simulink model "group5_A2finalmodel"  (R2023a)
settings: Solver=FixedStepAuto  StartTime=0.0  StopTime=10.0  FixedStep=1e-3  RelTol=1e-3  EnableMultiTasking=on
undefined symbols (not defined in the file): A0, A1, D0, D1, D10, D11, D12, D13, D2, D3, D4, D5, D6, D7, D8, D9, PTA0, PTA1, PTA2, PTB2, PTB23, PTB3, PTB9, PTC16, PTC17, PTC2, PTC3, PTC4, PTD0, PTD1, PTD2, PTD3
libraries: frdmk64flib x19, etargetslib x4, dspstat3 x1
settings Model: ExtModeTrigDuration=5  Creator=josep  LastModifiedBy=alast
settings SolverCC: AlgebraicLoopSolver=TrustRegion
settings OptimizationCC: EnhancedBackFolding=on  PassReuseOutputArgsAs=Individual arguments  ZeroExternalMemoryAtStartup=off  ZeroInternalMemoryAtStartup=off  MaxStackSize=64  OptimizeBlockOrder=speed  DifferentSizesBufferReuse=on  OptimizationCustomize=off  EfficientTunableParamExpr=on
settings DebuggingCC: ParameterTunabilityLossMsg=error
settings HardwareCC: ProdBitPerPointer=32  ProdBitPerSizeT=32  ProdBitPerPtrDiffT=32  ProdLargestAtomicInteger=Long  ProdLargestAtomicFloat=Double  ProdWordSize=32  ProdHWDeviceType=ARM Compatible->ARM Cortex
settings SFSimCC: MATLABDynamicMemAlloc=off
settings RTWCC: Description=Embedded Coder  SystemTargetFile=ert.tlc  HardwareBoard=NXP FRDM-K64F  TLCOptions="-aInlineSetEventsForThisBaseRateFcn=TLC_FALSE -aSuppressMultiTaskScheduler=TLC_FALSE  -aRateBasedStepFcn=0"  TemplateMakefile=ert_default_tmf  Toolchain=GNU Tools for ARM Embedded Processors
settings CodeAppCC: ForceParamTrailComments=on  IgnoreCustomStorageClasses=off  OperatorAnnotations=on  SimulinkDataObjDesc=on  SFDataObjDesc=on  InsertBlockDesc=on
settings ERTTargetCC: ExtModeTransport=4  ExtModeMexFile=sendToCommService

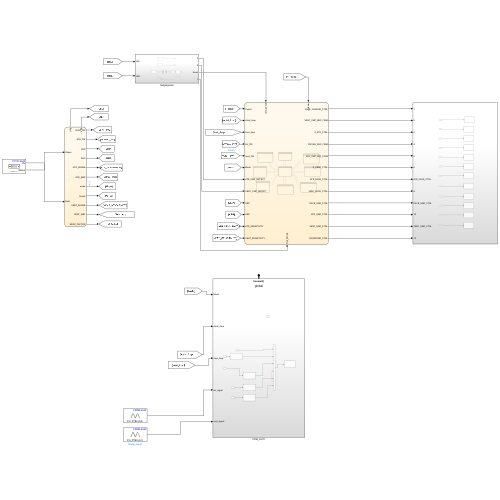
[thumbnail: Simulink's stored preview of the top-level diagram]
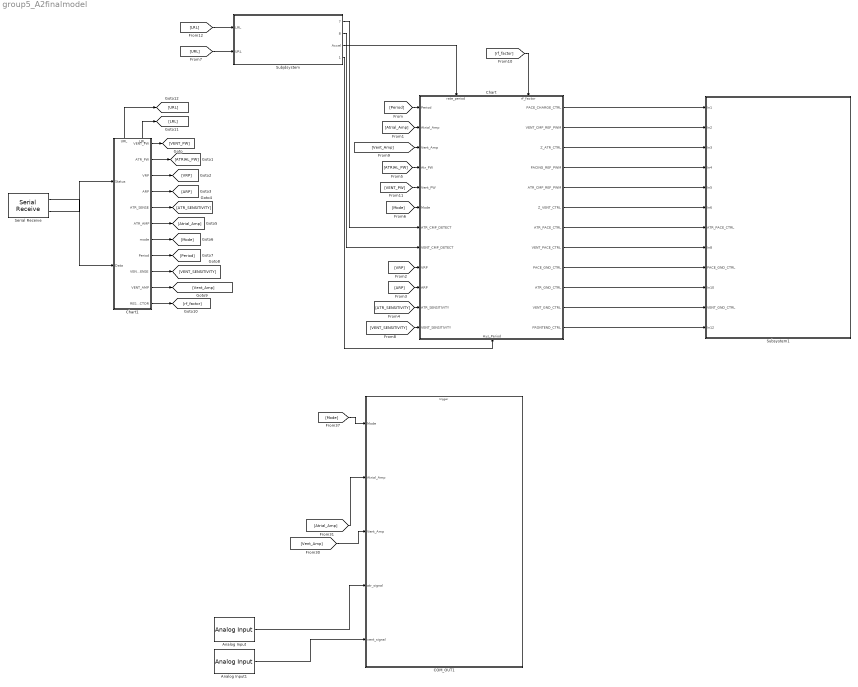
== system group5_A2finalmodel ==
  Analog Input : frdmk64flib/Analog Input  Whichpin=PTB2 (A0)  SampleTime=-1
  Analog Input1 : frdmk64flib/Analog Input  Whichpin=PTB3 (A1)  SampleTime=-1
  COM_OUT1 : Subsystem  TreatAsAtomicUnit=on
  Chart : Stateflow chart  TreatAsAtomicUnit=on
      settings: PortSchema="{\"entries\":[{\"content\":{\"sides\":[{\"content\":{\"connectorIds\":[\"In8\",\"In4\",\"In5\",\"In6\",\"In7\",\"In9\",\"In10\",\"In11\",\"In12\",\"In13\",\"In14\",\"In15\"]},\"type\":\"ConnectorPlacement.EquallySpacedRectSide\",\"uuid\":\"6343ef83-1ce8-46c7-8622-1dca0f09a909\"},{\"content\":{\"connectorIds\":[\"Out1\",\"Out2\",\"Out3\",\"Out4\",\"Out5\",\"Out6\",\"Out7\",\"Out8\",\"Out9\",\"Out10\",\"Out11\",\"Out12\"],\"side\":\"RIGHT\"},\"type\":\"ConnectorPlacement.EquallySpacedRectSide\",\"uuid\":\"7d8c9973-a2ea-42d1-99a2-efee47476445\"},{\"content\":{\"connectorIds\":[\"In1\",\"In2\"],\"side\":\"TOP\"},\"type\":\"ConnectorPlacement.EquallySpacedRectSide\",\"uuid\":\"d6f36041-fe62-4fd0-b92e-ddcbd2ff161d\"},{\"content\":{\"connectorIds\":[\"In3\"],\"side\":\"BOTTOM\"},\"type\":\"ConnectorPlacement.EquallySpacedRectSide\",\"uuid\":\"9ef693f9-8331-444a-9668-ba4dbf8aea62\"}]},\"type\":\"ConnectorPlacement.EquallySpacedConnector\",\"uuid\":\"1488a652-70a0-4b94-9610-167d4f46302b\"}],\"packageUris\":[\"http://schema.mathworks.com/mf0/Connector/R2020b\"],\"version\":\"1.0\"}"
  Chart1 : Stateflow chart  TreatAsAtomicUnit=on
      settings: PortSchema="{\"entries\":[{\"content\":{\"sides\":[{\"content\":{\"connectorIds\":[\"In1\",\"In2\"]},\"type\":\"ConnectorPlacement.EquallySpacedRectSide\",\"uuid\":\"8fb2c45e-5549-4401-9c79-42eba0e918c6\"},{\"content\":{\"connectorIds\":[\"Out3\",\"Out4\",\"Out5\",\"Out6\",\"Out7\",\"Out8\",\"Out9\",\"Out10\",\"Out11\",\"Out12\",\"Out13\"],\"side\":\"RIGHT\"},\"type\":\"ConnectorPlacement.EquallySpacedRectSide\",\"uuid\":\"7f0c3680-1cc1-4ed2-8a94-80b3abd25fe2\"},{\"content\":{\"connectorIds\":[\"Out1\",\"Out2\"],\"side\":\"TOP\"},\"type\":\"ConnectorPlacement.EquallySpacedRectSide\",\"uuid\":\"e6a4cd4f-b629-40f1-b56f-49c003080cda\"}]},\"type\":\"ConnectorPlacement.EquallySpacedConnector\",\"uuid\":\"c978f693-ab67-4a6f-917b-57d5c3fb90c1\"}],\"packageUris\":[\"http://schema.mathworks.com/mf0/Connector/R2020b\"],\"version\":\"1.0\"}"
  Serial Receive : frdmk64flib/Serial Receive  SCIModule=0  Baudrate=uint32(9600)  Parity=None  StopBits=1  HardwareFlowControl=None  ByteOrder=LittleEndian  DataType=uint8  DataLength=34  BlockingMode=off  OutputStatus=on  SampleTime=-1
  Subjdsystem : Subsystem
  Subsystem1 : Subsystem
  wires:
  Subjdsystem/1(7) -> Chart/10(ATR_CMP_DETECT)
  Subjdsystem/2(8) -> Chart/11(VENT_CMP_DETECT)
  Subjdsystem/3(Accel) -> Chart/1(rate_period)
  Chart/6(Z_VENT_CTRL) -> Subsystem1/6(In6)
  Chart/5(ATR_CMP_REF_PWM) -> Subsystem1/5(In5)
  Chart/4(PACING_REF_PWM) -> Subsystem1/4(In4)
  Chart/3(Z_ATR_CTRL) -> Subsystem1/3(In3)
  Chart/2(VENT_CMP_REF_PWM) -> Subsystem1/2(In2)
  Chart/7(ATR_PACE_CTRL) -> Subsystem1/7(ATR_PACE_CTRL)
  Chart/8(VENT_PACE_CTRL) -> Subsystem1/8(In8)
  Chart/9(PACE_GND_CTRL) -> Subsystem1/9(PACE_GND_CTRL)
  Chart/10(ATR_GND_CTRL) -> Subsystem1/10(In10)
  Chart/11(VENT_GND_CTRL) -> Subsystem1/11(VENT_GND_CTRL)
  Chart/12(FRONTEND_CTRL) -> Subsystem1/12(In12)
  Chart/1(PACE_CHARGE_CTRL) -> Subsystem1/1(In1)
  Subjdsystem/4(1) -> Chart/3(Hys_Period)
  Serial Receive/1 -> Chart1/2(Data)
  Serial Receive/2 -> Chart1/1(Status)
  [Atrial_Amp] -> COM_OUT1/2(Atrial_Amp)
  [Vent_Amp] -> COM_OUT1/3(Vent_Amp)
  [Mode] -> COM_OUT1/1(Mode)
  Chart1/3(VENT_PW) -> [VENT_PW]
  Chart1/4(ATR_PW) -> [ATRIAL_PW]
  Chart1/5(VRP) -> [VRP]
  Chart1/6(ARP) -> [ARP]
  Chart1/7(ATR_SENSE) -> [ATR_SENSITIVITY]
  Chart1/8(ATR_AMP) -> [Atrial_Amp]
  Chart1/9(mode) -> [Mode]
  Chart1/10(Period) -> [Period]
  Chart1/11(VENT_SENSE) -> [VENT_SENSITIVITY]
  Chart1/12(VENT_AMP) -> [Vent_Amp]
  Chart1/13(RESP_FACTOR) -> [rf_factor]
  [Period] -> Chart/8(Period)
  [Atrial_Amp] -> Chart/4(Atrial_Amp)
  [VRP] -> Chart/12(VRP)
  [ARP] -> Chart/13(ARP)
  [ATR_SENSITIVITY] -> Chart/14(ATR_SENSITIVITY)
  [VENT_SENSITIVITY] -> Chart/15(VENT_SENSITIVITY)
  [ATRIAL_PW] -> Chart/6(Atr_PW)
  [VENT_PW] -> Chart/7(Vent_PW)
  [Mode] -> Chart/9(Mode)
  [Vent_Amp] -> Chart/5(Vent_Amp)
  [rf_factor] -> Chart/2(rf_factor)
  Analog Input/1 -> COM_OUT1/4(atr_signal)
  Analog Input1/1 -> COM_OUT1/5(vent_signal)
  Chart1/2(LRL) -> [LRL]
  Chart1/1(URL) -> [URL]
  [URL] -> Subjdsystem/2(URL)
  [LRL] -> Subjdsystem/1(LRL)

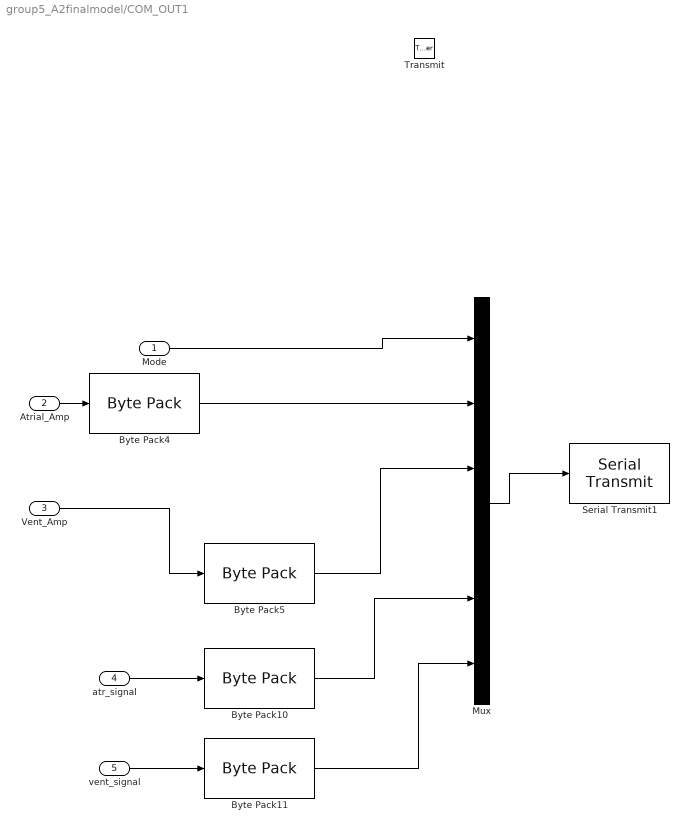
== system group5_A2finalmodel/COM_OUT1 ==
  Mode : Inport
  Atrial_Amp : Inport  Port=2
  Vent_Amp : Inport  Port=3
  atr_signal : Inport  Port=4
  vent_signal : Inport  Port=5
  Transmit : TriggerPort  TriggerType=function-call  IsSimulinkFunction=on  FunctionName=transmit  VariantControl=Variant
  Byte Pack10 : etargetslib/Byte Pack  datatypes={'double'}  byteAlign=1
  Byte Pack11 : etargetslib/Byte Pack  datatypes={'double'}  byteAlign=1
  Byte Pack4 : etargetslib/Byte Pack  datatypes={'single'}  byteAlign=1
  Byte Pack5 : etargetslib/Byte Pack  datatypes={'single'}  byteAlign=1
  Mux : Mux  Inputs=6
  Serial Transmit1 : frdmk64flib/Serial Transmit  SCIModule=0  Baudrate=uint32(9600)  Parity=None  StopBits=1  HardwareFlowControl=None  ByteOrder=LittleEndian  BlockingMode=on  OutputStatus=off
  wires:
  Mode/1 -> Mux/1
  Mux/1 -> Serial Transmit1/1
  Atrial_Amp/1 -> Byte Pack4/1
  Byte Pack4/1 -> Mux/2
  Vent_Amp/1 -> Byte Pack5/1
  Byte Pack5/1 -> Mux/3
  atr_signal/1 -> Byte Pack10/1
  Byte Pack10/1 -> Mux/5
  vent_signal/1 -> Byte Pack11/1
  Byte Pack11/1 -> Mux/6
  ? -> Mux/4

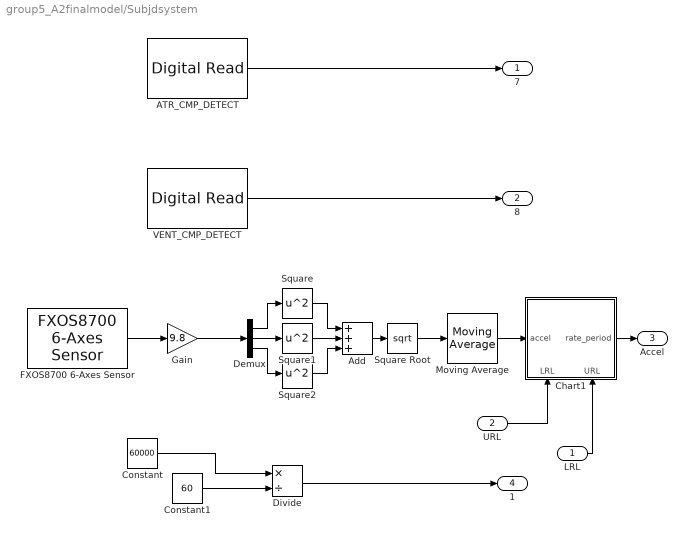
== system group5_A2finalmodel/Subjdsystem ==
  LRL : Inport
  URL : Inport  Port=2
  ATR_CMP_DETECT : frdmk64flib/Digital Read  Whichpin=PTC16 (D0)  SampleTime=-1
  Add : Sum  Inputs=+++
  Chart1 : Stateflow chart  TreatAsAtomicUnit=on
      settings: PortSchema="{\"entries\":[{\"content\":{\"sides\":[{\"content\":{\"connectorIds\":[\"In3\"]},\"type\":\"ConnectorPlacement.EquallySpacedRectSide\",\"uuid\":\"e23e5e59-a455-450d-92cc-53adb6a0dadc\"},{\"content\":{\"connectorIds\":[\"Out1\"],\"side\":\"RIGHT\"},\"type\":\"ConnectorPlacement.EquallySpacedRectSide\",\"uuid\":\"9f1d0732-5dc7-42dd-8692-2a9a32444121\"},{\"content\":{\"connectorIds\":[],\"side\":\"TOP\"},\"type\":\"ConnectorPlacement.EquallySpacedRectSide\",\"uuid\":\"ad335b18-86a7-4912-8815-32b944d46f48\"},{\"content\":{\"connectorIds\":[\"In1\",\"In2\"],\"side\":\"BOTTOM\"},\"type\":\"ConnectorPlacement.EquallySpacedRectSide\",\"uuid\":\"4746a105-19d6-4e83-8176-b66af7bc6762\"}]},\"type\":\"ConnectorPlacement.EquallySpacedConnector\",\"uuid\":\"39913b06-9f7c-4388-b951-2bea9bac005b\"}],\"packageUris\":[\"http://schema.mathworks.com/mf0/Connector/19700101\"],\"version\":\"1.0\"}"
  Constant : Constant  Value=60000
  Constant1 : Constant  Value=60
  Demux : Demux  Outputs=3
  Divide : Product  Inputs=*/
  FXOS8700 6-Axes Sensor : frdmk64flib/FXOS8700 6-Axes Sensor  Activesensor=Accelerometer only  ODR=800Hz  HybridODR=400Hz  Accelfullrange=-4g to +4g  SampleTime=-1
  Gain : Gain  Gain=9.8
  Moving Average : dspstat3/Moving Average  Method=Sliding window  ForgettingFactorPort=off  SpecifyWindowLength=on  WindowLength=4  OverlapLength=3  AllowArbitraryInputLength=off  ForgettingFactor=0.9  SimulateUsing=Code generation
  Square : Math  Operator=square
  Square Root : Sqrt
  Square1 : Math  Operator=square
  Square2 : Math  Operator=square
  VENT_CMP_DETECT : frdmk64flib/Digital Read  Whichpin=PTC17 (D1)  SampleTime=-1
  7 : Outport
  8 : Outport  Port=2
  Accel : Outport  Port=3
  1 : Outport  Port=4
  wires:
  ATR_CMP_DETECT/1 -> 7/1
  VENT_CMP_DETECT/1 -> 8/1
  Square/1 -> Add/1
  Demux/1 -> Square/1
  Add/1 -> Square Root/1
  Square2/1 -> Add/3
  Square Root/1 -> Moving Average/1
  FXOS8700 6-Axes Sensor/1 -> Gain/1
  Square1/1 -> Add/2
  Demux/2 -> Square1/1
  Gain/1 -> Demux/1
  Demux/3 -> Square2/1
  Chart1/1(rate_period) -> Accel/1
  Moving Average/1 -> Chart1/3(accel)
  Constant/1 -> Divide/1
  Constant1/1 -> Divide/2
  Divide/1 -> 1/1
  URL/1 -> Chart1/1(LRL)
  LRL/1 -> Chart1/2(URL)

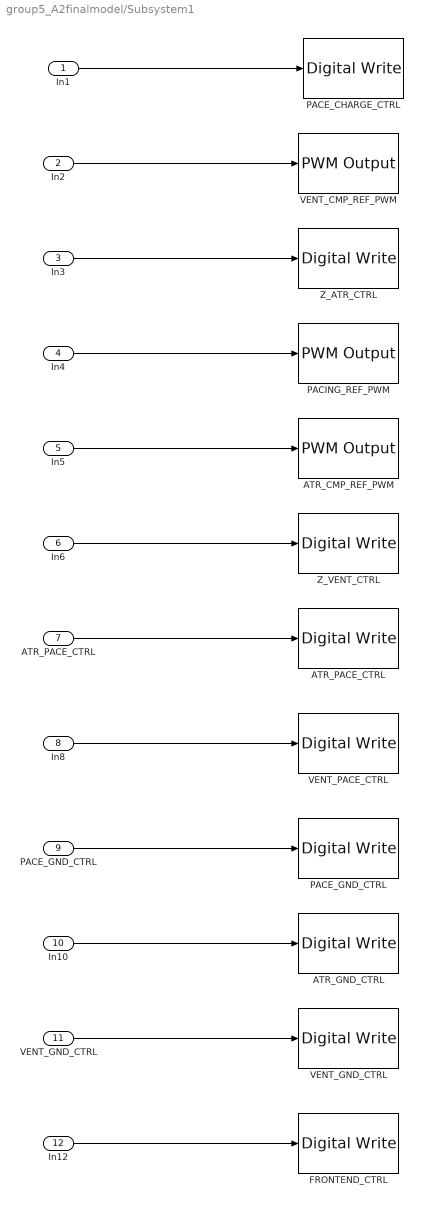
== system group5_A2finalmodel/Subsystem1 ==
  In1 : Inport
  In2 : Inport  Port=2
  In3 : Inport  Port=3
  In4 : Inport  Port=4
  In5 : Inport  Port=5
  In6 : Inport  Port=6
  ATR_PACE_CTRL : Inport  Port=7
  In8 : Inport  Port=8
  PACE_GND_CTRL : Inport  Port=9
  In10 : Inport  Port=10
  VENT_GND_CTRL : Inport  Port=11
  In12 : Inport  Port=12
  ATR_CMP_REF_PWM : frdmk64flib/PWM Output  Whichpin=PTC2 (D6)  InitialFrequency=2000  InitialDutyCycle=0
  ATR_GND_CTRL : frdmk64flib/Digital Write  Whichpin=PTD2 (D11)
  "ATR_PACE_CTRL " : frdmk64flib/Digital Write  Whichpin=PTA0 (D8)
  FRONTEND_CTRL : frdmk64flib/Digital Write  Whichpin=PTD1 (D13)
  PACE_CHARGE_CTRL : frdmk64flib/Digital Write  Whichpin=PTB9 (D2)
  "PACE_GND_CTRL " : frdmk64flib/Digital Write  Whichpin=PTD0 (D10)
  PACING_REF_PWM : frdmk64flib/PWM Output  Whichpin=PTA2 (D5)  InitialFrequency=2000  InitialDutyCycle=0
  VENT_CMP_REF_PWM : frdmk64flib/PWM Output  Whichpin=PTA1 (D3)  InitialFrequency=2000  InitialDutyCycle=0
  "VENT_GND_CTRL " : frdmk64flib/Digital Write  Whichpin=PTD3 (D12)
  VENT_PACE_CTRL : frdmk64flib/Digital Write  Whichpin=PTC4 (D9)
  Z_ATR_CTRL : frdmk64flib/Digital Write  Whichpin=PTB23 (D4)
  Z_VENT_CTRL : frdmk64flib/Digital Write  Whichpin=PTC3 (D7)
  wires:
  In1/1 -> PACE_CHARGE_CTRL/1
  In2/1 -> VENT_CMP_REF_PWM/1
  In3/1 -> Z_ATR_CTRL/1
  In4/1 -> PACING_REF_PWM/1
  In5/1 -> ATR_CMP_REF_PWM/1
  In6/1 -> Z_VENT_CTRL/1
  ATR_PACE_CTRL/1 -> "ATR_PACE_CTRL "/1
  In8/1 -> VENT_PACE_CTRL/1
  In12/1 -> FRONTEND_CTRL/1
  PACE_GND_CTRL/1 -> "PACE_GND_CTRL "/1
  VENT_GND_CTRL/1 -> "VENT_GND_CTRL "/1
  In10/1 -> ATR_GND_CTRL/1

== stateflow chart group5_A2finalmodel/Subjdsystem/Chart1 ==
  state Resting1
    rate_period=60000/Lowest;
  state Rest_Mid1
    rate_period= 60000/(Lowest+Interval);
  state initial1
    entry:
    Lowest=LRL;
    Highest=URL;
    Interval=(URL-LRL)/4;
  state Mid1
    rate_period = 60000/(Lowest+Interval+Interval);
  state Resting [commented out]
    rate_period=60000/70;
  state Mid_high1
    rate_period = (60000/Lowest+Interval+Interval+Interval);
  state High1
    rate_period=(60000/Highest);
  state Rest_Mid [commented out]
    rate_period= 60000/92.5;
  state initial [commented out]
  state Mid [commented out]
    rate_period = 60000/115;
  state Mid_high [commented out]
    rate_period = 60000/137.5;
  state High [commented out]
    rate_period=60000/160;
  Resting1 -> initial1
  initial1 -> Resting1 [order 2] : [accel <11]
  (default) -> initial1
  initial1 -> Rest_Mid1 [order 3] : [accel >=11 && accel < 22]
  Rest_Mid1 -> initial1
  initial1 -> Mid1 [order 5] : [accel >=22 && accel <33]
  Mid1 -> initial1
  High1 -> initial1
  initial1 -> High1 [order 1] : [accel>=44]
  Mid_high1 -> initial1
  initial1 -> Mid_high1 [order 4] : [accel>=33 && accel < 44]
  Resting -> initial [commented out]
  initial -> Resting [commented out] : [accel <11]
  (default) -> initial [commented out]
  initial -> Rest_Mid [commented out] : [accel >=11 && accel < 22]
  Rest_Mid -> initial [commented out]
  initial -> Mid [commented out] : [accel >=22 && accel <33]
  Mid -> initial [commented out]
  High -> initial [commented out]
  initial -> High [commented out] : [accel>=44]
  Mid_high -> initial [commented out]
  initial -> Mid_high [commented out] : [accel>=33 && accel < 44]
  data: LRL input; URL input; accel input; rate_period output; Highest local; Lowest local; Interval local

== stateflow chart group5_A2finalmodel/Chart1 ==
  state Set_Param
    entry:
    mode = Data(2);
    Period = Data(3);
    ATR_AMP = typecast(Data(4:7),'single');
    VENT_AMP = typecast(Data(8:11),'single');
    ATR_PW = typecast(Data(12:15),'single');
    VENT_PW =typecast(Data(16:19),'single');
    ARP = typecast(Data(20:21),'uint16');
    VRP = typecast(Data(22:23),'uint16');
    ATR_SENSE = typecast(Data(24:27),'single');
    VENT_SENSE = typecast(Data(28:31),'single');
    RESP_FACTOR =Data(32);
    URL = Data(33);
    LRL = Data(34);
  state Initial
    entry:
    mode = 1;
    Period = 80;
    ATR_AMP = 1.0;
    VENT_AMP = 1.0;
    ATR_PW = 0.5;
    VENT_PW = 0.5;
    ARP = 400;
    VRP = 500;
    ATR_SENSE = 0.25;
    VENT_SENSE = 0.25;
    RESP_FACTOR =4;
    LRL = 60;
    URL = 160;
  state Standby
  state Echo
    entry:
    transmit();
  (default) -> Initial
  Set_Param -> Standby
  Initial -> Standby
  Echo -> Standby
  Standby -> (junction 39) : [Status ==0]
  (junction 39) -> Set_Param [order 1] : [Data(1) == 1]
  (junction 39) -> Echo [order 2] : [Data(1) == 0]
  data: URL output uint8; LRL output uint8; Status input uint8; Data input uint8; VENT_PW output single; ATR_PW output single; VRP output uint16; ARP output uint16; ATR_SENSE output single; ATR_AMP output single; mode output uint8; Period output uint8; VENT_SENSE output single; VENT_AMP output single; RESP_FACTOR output uint8

== stateflow chart group5_A2finalmodel/Chart ==
  state VOOR
    state decrease
      entry:
      copy_Period = copy_Period-single(rf_factor);
    state increase
      entry:
      copy_Period = copy_Period+single(rf_factor);
    state Initate
      entry:
      copy_Period = single(Period)
    state Charging
      entry:
      %Charging C22
      ATR_PACE_CTRL = 0
      VENT_PACE_CTRL = 0
      PACING_REF_PWM = Vent_Amp
      PACE_CHARGE_CTRL = 1
      %Discharging C21
      PACE_GND_CTRL = 1
      VENT_PACE_CTRL = 0
      Z_ATR_CTRL = 0
      Z_VENT_CTRL = 0
      ATR_PACE_CTRL = 0
      ATR_GND_CTRL = 0
      VENT_GND_CTRL = 1
    state Discharging
      entry:
      %Discharge C22 into C21
      PACE_CHARGE_CTRL = 0
      PACE_GND_CTRL = 1
      ATR_PACE_CTRL = 0
      ATR_GND_CTRL = 0
      Z_VENT_CTRL = 0
      Z_ATR_CTRL = 0
      VENT_GND_CTRL = 0
      VENT_PACE_CTRL = 1
    VOOR.decrease -> VOOR.Charging : [after(Vent_PW, msec)]
    VOOR.Discharging -> VOOR.decrease [order 2] : [copy_Period>rate_period]
    (default) -> VOOR.Initate
    VOOR.increase -> VOOR.Charging : [after(Vent_PW, msec)]
    VOOR.Initate -> VOOR.Charging
    VOOR.Discharging -> VOOR.increase [order 1] : [copy_Period<rate_period]
    (junction 284) -> VOOR.Charging : [after(Vent_PW, msec)]
    VOOR.Discharging -> (junction 284) [order 3] : [copy_Period==rate_period]
    VOOR.Charging -> VOOR.Discharging : [after(single(copy_Period) - Vent_PW, msec)]
  state VOO
    state Discharging
      entry:
      %Discharge C22 into C21
      PACE_CHARGE_CTRL = 0
      PACE_GND_CTRL = 1
      ATR_PACE_CTRL = 0
      ATR_GND_CTRL = 0
      Z_VENT_CTRL = 0
      Z_ATR_CTRL = 0
      VENT_GND_CTRL = 0
      VENT_PACE_CTRL = 1
    state Charging
      entry:
      %Charging C22
      ATR_PACE_CTRL = 0
      VENT_PACE_CTRL = 0
      PACING_REF_PWM = Vent_Amp
      PACE_CHARGE_CTRL = 1
      %Discharging C21
      PACE_GND_CTRL = 1
      VENT_PACE_CTRL = 0
      Z_ATR_CTRL = 0
      Z_VENT_CTRL = 0
      ATR_PACE_CTRL = 0
      ATR_GND_CTRL = 0
      VENT_GND_CTRL = 1
    (default) -> VOO.Charging
    VOO.Discharging -> VOO.Charging : [[after(Vent_PW, msec)]]
    VOO.Charging -> VOO.Discharging : [[after(single(Period) - Vent_PW, msec)]]
  state AOOR
    state decrease
      entry:
      copy_Period = copy_Period-single(rf_factor);
    state increase
      entry:
      copy_Period = copy_Period+single(rf_factor);
    state Initate
      entry:
      copy_Period = single(Period)
    state Charging
      entry:
      % Charging C22
      ATR_PACE_CTRL = 0
      VENT_PACE_CTRL = 0
      PACING_REF_PWM = Atrial_Amp
      PACE_CHARGE_CTRL = 1
      %  Discharge C21 while
      PACE_GND_CTRL = 1
      ATR_PACE_CTRL = 0
      Z_ATR_CTRL = 0
      Z_VENT_CTRL = 0
      ATR_GND_CTRL = 1
      VENT_GND_CTRL = 0
      VENT_PACE_CTRL = 0
    state Pacing
      entry:
      % Discharging C22 to C21
      PACE_CHARGE_CTRL = 0
      PACE_GND_CTRL = 1
      VENT_PACE_CTRL = 0
      Z_ATR_CTRL = 0
      Z_VENT_CTRL = 0
      ATR_PACE_CTRL = 1
      ATR_GND_CTRL = 0
      VENT_GND_CTRL = 0
    AOOR.decrease -> AOOR.Charging : [after(Atr_PW, msec)]
    AOOR.Pacing -> AOOR.decrease [order 3] : [copy_Period>rate_period]
    (default) -> AOOR.Initate
    AOOR.increase -> AOOR.Charging : [after(Atr_PW, msec)]
    AOOR.Pacing -> AOOR.increase [order 2] : [copy_Period<rate_period]
    AOOR.Initate -> AOOR.Charging
    AOOR.Pacing -> (junction 281) [order 1] : [copy_Period==rate_period]
    (junction 281) -> AOOR.Charging : [after(Atr_PW, msec)]
    AOOR.Charging -> AOOR.Pacing : [after(single(copy_Period) - Atr_PW, msec)]
  state AAI
    note: not sure why but dont subtract arp
    state Pacing
      entry:
      % Discharging C22 to C21
      PACE_CHARGE_CTRL = 0
      PACE_GND_CTRL = 1
      VENT_PACE_CTRL = 0
      Z_ATR_CTRL = 0
      Z_VENT_CTRL = 0
      ATR_PACE_CTRL = 1
      ATR_GND_CTRL = 0
      VENT_GND_CTRL = 0
      %ARP ON
      Set_ARP=1
    state Charging_sensing
      entry:
      %Sensing on
      FRONTEND_CTRL = 1
      ATR_CMP_REF_PWM = ATR_SENSITIVITY
      % Charging C22
      ATR_PACE_CTRL = 0
      VENT_PACE_CTRL = 0
      PACING_REF_PWM = Atrial_Amp
      PACE_CHARGE_CTRL = 1
      %  Discharge C21 while
      PACE_GND_CTRL = 1
      ATR_PACE_CTRL = 0
      Z_ATR_CTRL = 0
      Z_VENT_CTRL = 0
      ATR_GND_CTRL = 1
      VENT_GND_CTRL = 0
      VENT_PACE_CTRL = 0
    state INIT
      entry:
      Set_ARP=0
    state ARP_ON
      entry:
      Set_ARP=1
    (default) -> AAI.INIT
    AAI.Pacing -> AAI.Charging_sensing : [after(Atr_PW, msec)]
    (junction 256) -> AAI.Pacing [order 1] : [after(single(Period)-Atr_PW, msec)]
    AAI.Charging_sensing -> (junction 254) [order 1] : [Set_ARP==1]
    (junction 254) -> (junction 256) : [after(ARP,msec)]
    AAI.INIT -> AAI.Charging_sensing
    (junction 256) -> AAI.ARP_ON [order 2] : [ATR_CMP_DETECT==1]
    AAI.ARP_ON -> AAI.Charging_sensing
    (junction 247) -> AAI.ARP_ON [order 1] : [ATR_CMP_DETECT==1]
    (junction 247) -> AAI.Pacing [order 2] : [after(single(Period)-Atr_PW, msec)]
    AAI.Charging_sensing -> (junction 247) [order 2] : [Set_ARP==0]
  state Mode_Start
  state AOO
    state Charging
      entry:
      % Charging C22
      ATR_PACE_CTRL = 0
      VENT_PACE_CTRL = 0
      PACING_REF_PWM = Atrial_Amp
      PACE_CHARGE_CTRL = 1
      %  Discharge C21 while
      PACE_GND_CTRL = 1
      ATR_PACE_CTRL = 0
      Z_ATR_CTRL = 0
      Z_VENT_CTRL = 0
      ATR_GND_CTRL = 1
      VENT_GND_CTRL = 0
      VENT_PACE_CTRL = 0
    state Pacing
      entry:
      % Discharging C22 to C21
      PACE_CHARGE_CTRL = 0
      PACE_GND_CTRL = 1
      VENT_PACE_CTRL = 0
      Z_ATR_CTRL = 0
      Z_VENT_CTRL = 0
      ATR_PACE_CTRL = 1
      ATR_GND_CTRL = 0
      VENT_GND_CTRL = 0
    (default) -> AOO.Charging
    AOO.Pacing -> AOO.Charging : [after(Atr_PW, msec)]
    AOO.Charging -> AOO.Pacing : [after(single(Period) - Atr_PW, msec)]
  state DDDR [commented out]
    state rate_adjust4 [commented out]
      state decrease2 [commented out]
        entry:
        copy_Period = copy_Period-50
      state increase2 [commented out]
        entry:
        copy_Period = copy_Period+50
      (junction 880) -> DDDR.rate_adjust4.decrease2 [commented out] : [copy_Period>rate_period]
      DDDR.rate_adjust4.decrease2 -> (junction 881) [commented out]
      (junction 880) -> (junction 881) [commented out] : [copy_Period==rate_period]
      (junction 880) -> DDDR.rate_adjust4.increase2 [commented out] : [copy_Period<rate_period]
      DDDR.rate_adjust4.increase2 -> (junction 881) [commented out]
    state Rate_adjust [commented out]
      state decrease [commented out]
        entry:
        copy_Period = copy_Period-50
      state increase [commented out]
        entry:
        copy_Period = copy_Period+50
      DDDR.Rate_adjust.decrease -> DDDR.Rate_adjust [commented out]
      DDDR.Rate_adjust.increase -> DDDR.Rate_adjust [commented out]
    state Discharging [commented out]
      entry:
      %Discharge C22 into C21
      PACE_CHARGE_CTRL = 0
      PACE_GND_CTRL = 1
      Z_VENT_CTRL = 0
      Z_ATR_CTRL = 0
      VENT_GND_CTRL = 0
      VENT_PACE_CTRL = 1
      %test
      ATR_GND_CTRL=1
    state rate_adjust [commented out]
      state decrease2 [commented out]
        entry:
        copy_Period = copy_Period-single(rf_factor);
      state increase2 [commented out]
        entry:
        copy_Period = copy_Period+single(rf_factor);
      (junction 898) -> DDDR.rate_adjust.decrease2 [commented out] : [copy_Period>single(rate_period)]
      DDDR.rate_adjust.decrease2 -> (junction 899) [commented out]
      (junction 898) -> (junction 899) [commented out] : [copy_Period==single(rate_period)]
      (junction 898) -> DDDR.rate_adjust.increase2 [commented out] : [copy_Period<single(rate_period)]
      DDDR.rate_adjust.increase2 -> (junction 899) [commented out]
    state Pacing1 [commented out]
      entry:
      % Discharging C22 to C21
      PACE_CHARGE_CTRL = 0
      PACE_GND_CTRL = 1
      VENT_PACE_CTRL = 0
      Z_ATR_CTRL = 0
      Z_VENT_CTRL = 0
      ATR_PACE_CTRL = 1
      ATR_GND_CTRL = 0
      VENT_GND_CTRL = 0
      %ARP ON
      Set_ARP=1
      Hys=0
    state Charging_sensing1 [commented out]
      entry:
      %Sensing on
      FRONTEND_CTRL = 1
      ATR_CMP_REF_PWM = ATR_SENSITIVITY
      % Charging C22
      ATR_PACE_CTRL = 0
      VENT_PACE_CTRL = 0
      PACING_REF_PWM = Atrial_Amp
      PACE_CHARGE_CTRL = 1
      %  Discharge C21 while
      PACE_GND_CTRL = 1
      ATR_PACE_CTRL = 0
      Z_ATR_CTRL = 0
      Z_VENT_CTRL = 0
      ATR_GND_CTRL = 1
      VENT_GND_CTRL = 0
      VENT_PACE_CTRL = 0
    state INIT1 [commented out]
      entry:
      Set_ARP=0
      copy_Period=Period
      Hys=0
    note: Hys_on is an input data (locally set for testing)
    state INIT [commented out]
      entry:
      Set_ARP=0
      copy_Period=single(Period)
      Hys=0
      Hys_delay=Hys_Period
      Hys_on=0
      AV_delay=180
      A_Amp=Atrial_Amp
    state hys_check [commented out]
      (junction 915) -> (junction 916) [commented out] : [Hys==1]
      (junction 915) -> ? [commented out] : [Hys==0]
      (junction 916) -> ? [commented out]
    state ARP_ON1 [commented out]
      entry:
      Set_ARP=1
      Hys=1
    state rate_adjust3 [commented out]
      state decrease2 [commented out]
        entry:
        copy_Period = copy_Period-50
      state increase2 [commented out]
        entry:
        copy_Period = copy_Period+50
      (junction 925) -> DDDR.rate_adjust3.decrease2 [commented out] : [copy_Period>rate_period]
      DDDR.rate_adjust3.decrease2 -> (junction 926) [commented out]
      (junction 925) -> (junction 926) [commented out] : [copy_Period==rate_period]
      (junction 925) -> DDDR.rate_adjust3.increase2 [commented out] : [copy_Period<rate_period]
      DDDR.rate_adjust3.increase2 -> (junction 926) [commented out]
    state Charging_sensing [commented out]
      entry:
      % Charging C22
      ATR_PACE_CTRL = 0
      VENT_PACE_CTRL = 0
      PACING_REF_PWM = A_Amp
      PACE_CHARGE_CTRL = 1
      %  Discharge C21 while
      PACE_GND_CTRL = 1
      ATR_PACE_CTRL = 0
      Z_ATR_CTRL = 0
      Z_VENT_CTRL = 0
      ATR_GND_CTRL = 1
      VENT_GND_CTRL = 1
      ATR_CMP_REF_PWM = ATR_SENSITIVITY
    state charging [commented out]
      entry:
      %Charging C22
      ATR_PACE_CTRL = 0
      VENT_PACE_CTRL = 0
      PACING_REF_PWM = A_Amp
      PACE_CHARGE_CTRL = 1
      %  Discharge C21 while
      PACE_GND_CTRL = 1
      Z_ATR_CTRL = 0
      Z_VENT_CTRL = 0
      ATR_GND_CTRL = 1
      VENT_GND_CTRL = 1
    state PacingATR [commented out]
      entry:
      % Discharging C22 to C21
      PACE_CHARGE_CTRL = 0
      PACE_GND_CTRL = 1
      Z_ATR_CTRL = 0
      Z_VENT_CTRL = 0
      ATR_PACE_CTRL = 1
      ATR_GND_CTRL = 0
      %test
      VENT_GND_CTRL = 1
    state rate_adjust5 [commented out]
      state decrease2 [commented out]
        entry:
        copy_Period = copy_Period-rf_factor;
      state increase2 [commented out]
        entry:
        copy_Period = copy_Period+rf_factor;
      (junction 940) -> DDDR.rate_adjust5.decrease2 [commented out] : [copy_Period>rate_period]
      DDDR.rate_adjust5.decrease2 -> (junction 941) [commented out]
      (junction 940) -> (junction 941) [commented out] : [copy_Period==rate_period]
      (junction 940) -> DDDR.rate_adjust5.increase2 [commented out] : [copy_Period<rate_period]
      DDDR.rate_adjust5.increase2 -> (junction 941) [commented out]
    PacingATR -> (junction 940) [commented out] : [Button==1]
    DDDR.Pacing1 -> (junction 880) [commented out] : [after(Atr_PW, msec)]
    (junction 881) -> DDDR.Charging_sensing1 [commented out]
    (default) -> DDDR.Rate_adjust.decrease [commented out] : [copy_Period>rate_period]
    (default) -> DDDR.Rate_adjust.increase [commented out] : [copy_Period<rate_period]
    (default) -> DDDR.Rate_adjust [commented out] : [copy_Period==rate_period]
    (default) -> DDDR.INIT1 [commented out]
    (junction 899) -> DDDR.Charging_sensing [commented out]
    (junction 926) -> DDDR.ARP_ON1 [commented out]
    (junction 941) -> DDDR.Charging_sensing [commented out]
    (junction 838) -> (junction 898) [commented out]
    (junction 841) -> DDDR.Discharging [commented out] : [Button==0]
    (default) -> DDDR.INIT [commented out]
    DDDR.Discharging -> (junction 838) [commented out]
    DDDR.INIT1 -> DDDR.Charging_sensing1 [commented out]
    (junction 840) -> DDDR.Pacing1 [commented out] : [after(copy_Period-Atr_PW ,msec)]
    (junction 841) -> (junction 838) [commented out] : [Button==1]
    DDDR.Charging_sensing1 -> (junction 839) [commented out] : [Set_ARP==1]
    (junction 839) -> (junction 840) [commented out] : [after(ARP,msec)]
    DDDR.ARP_ON1 -> DDDR.Charging_sensing1 [commented out]
    charging -> (junction 841) [commented out] : [after(AV_delay, msec)]
    (junction 842) -> DDDR.ARP_ON1 [commented out] : [ATR_CMP_DETECT==1]
    DDDR.INIT -> DDDR.Charging_sensing [commented out]
    DDDR.Charging_sensing1 -> (junction 842) [commented out] : [Set_ARP==0]
    (junction 842) -> DDDR.Pacing1 [commented out] : [after(copy_Period-Atr_PW, msec)]
    DDDR.Charging_sensing -> PacingATR [commented out] : [after((copy_Period-AV_delay),msec)]
    (junction 840) -> (junction 925) [commented out] : [ATR_CMP_DETECT==1]
    PacingATR -> charging [commented out]
  state AAIR
    state rate_adjust4 [commented out]
      state decrease2 [commented out]
        entry:
        copy_Period = copy_Period-50
      state increase2 [commented out]
        entry:
        copy_Period = copy_Period+50
      (junction 602) -> AAIR.rate_adjust4.decrease2 [commented out] : [copy_Period>rate_period]
      AAIR.rate_adjust4.decrease2 -> (junction 603) [commented out]
      (junction 602) -> (junction 603) [commented out] : [copy_Period==rate_period]
      (junction 602) -> AAIR.rate_adjust4.increase2 [commented out] : [copy_Period<rate_period]
      AAIR.rate_adjust4.increase2 -> (junction 603) [commented out]
    state Rate_adjust [commented out]
      state decrease [commented out]
        entry:
        copy_Period = copy_Period-50
      state increase [commented out]
        entry:
        copy_Period = copy_Period+50
      AAIR.Rate_adjust.decrease -> AAIR.Rate_adjust [commented out]
      AAIR.Rate_adjust.increase -> AAIR.Rate_adjust [commented out]
    state rate_adjust
      state decrease2
        entry:
        copy_Period = copy_Period-single(rf_factor)
      state increase2
        entry:
        copy_Period = copy_Period+single(rf_factor)
      (junction 455) -> AAIR.rate_adjust.decrease2 [order 1] : [copy_Period>rate_period]
      AAIR.rate_adjust.decrease2 -> (junction 461)
      (junction 455) -> (junction 461) [order 3] : [copy_Period==rate_period]
      (junction 455) -> AAIR.rate_adjust.increase2 [order 2] : [copy_Period<rate_period]
      AAIR.rate_adjust.increase2 -> (junction 461)
    state Pacing1 [commented out]
      entry:
      % Discharging C22 to C21
      PACE_CHARGE_CTRL = 0
      PACE_GND_CTRL = 1
      VENT_PACE_CTRL = 0
      Z_ATR_CTRL = 0
      Z_VENT_CTRL = 0
      ATR_PACE_CTRL = 1
      ATR_GND_CTRL = 0
      VENT_GND_CTRL = 0
      %ARP ON
      Set_ARP=1
      Hys=0
    state Charging_sensing1 [commented out]
      entry:
      %Sensing on
      FRONTEND_CTRL = 1
      ATR_CMP_REF_PWM = ATR_SENSITIVITY
      % Charging C22
      ATR_PACE_CTRL = 0
      VENT_PACE_CTRL = 0
      PACING_REF_PWM = Atrial_Amp
      PACE_CHARGE_CTRL = 1
      %  Discharge C21 while
      PACE_GND_CTRL = 1
      ATR_PACE_CTRL = 0
      Z_ATR_CTRL = 0
      Z_VENT_CTRL = 0
      ATR_GND_CTRL = 1
      VENT_GND_CTRL = 0
      VENT_PACE_CTRL = 0
    state INIT1 [commented out]
      entry:
      Set_ARP=0
      copy_Period=Period
      Hys=0
    note: Hys_on is an input data (locally set for testing)
    state hys_check [commented out]
      (junction 644) -> (junction 645) [commented out] : [Hys==1]
      (junction 644) -> ? [commented out] : [Hys==0]
      (junction 645) -> ? [commented out]
    state INIT
      entry:
      Set_ARP=0
      copy_Period=single(Period)
      Hys=0
      Hys_delay=Hys_Period
      Hys_on=1
    state ARP_ON1 [commented out]
      entry:
      Set_ARP=1
      Hys=1
    state rate_adjust3 [commented out]
      state decrease2 [commented out]
        entry:
        copy_Period = copy_Period-50
      state increase2 [commented out]
        entry:
        copy_Period = copy_Period+50
      (junction 589) -> AAIR.rate_adjust3.decrease2 [commented out] : [copy_Period>rate_period]
      AAIR.rate_adjust3.decrease2 -> (junction 590) [commented out]
      (junction 589) -> (junction 590) [commented out] : [copy_Period==rate_period]
      (junction 589) -> AAIR.rate_adjust3.increase2 [commented out] : [copy_Period<rate_period]
      AAIR.rate_adjust3.increase2 -> (junction 590) [commented out]
    state Pacing
      entry:
      % Discharging C22 to C21
      PACE_CHARGE_CTRL = 0
      PACE_GND_CTRL = 1
      VENT_PACE_CTRL = 0
      Z_ATR_CTRL = 0
      Z_VENT_CTRL = 0
      ATR_PACE_CTRL = 1
      ATR_GND_CTRL = 0
      VENT_GND_CTRL = 0
      %ARP ON
      Set_ARP=1
      Hys=0
    state Charging_sensing
      entry:
      %Sensing on
      FRONTEND_CTRL = 1
      ATR_CMP_REF_PWM = ATR_SENSITIVITY
      % Charging C22
      ATR_PACE_CTRL = 0
      VENT_PACE_CTRL = 0
      PACING_REF_PWM = Atrial_Amp
      PACE_CHARGE_CTRL = 1
      %  Discharge C21 while
      PACE_GND_CTRL = 1
      ATR_PACE_CTRL = 0
      Z_ATR_CTRL = 0
      Z_VENT_CTRL = 0
      ATR_GND_CTRL = 1
      VENT_GND_CTRL = 0
      VENT_PACE_CTRL = 0
      Hys_delay=100 %obtained from srsVVI
    state Hys_ON
      entry:
      Hys=1
    state rate_adjust2
      state decrease2
        entry:
        copy_Period = copy_Period-single(rf_factor)
      state increase2
        entry:
        copy_Period = copy_Period+single(rf_factor)
      (junction 538) -> AAIR.rate_adjust2.decrease2 [order 1] : [copy_Period>rate_period]
      AAIR.rate_adjust2.decrease2 -> (junction 539)
      (junction 538) -> (junction 539) [order 3] : [copy_Period==rate_period]
      (junction 538) -> AAIR.rate_adjust2.increase2 [order 2] : [copy_Period<rate_period]
      AAIR.rate_adjust2.increase2 -> (junction 539)
    state ARP_ON
      entry:
      Set_ARP=1
    state rate_adjust1
      state decrease2
        entry:
        copy_Period = copy_Period-single(rf_factor)
      state increase2
        entry:
        copy_Period = copy_Period+single(rf_factor)
      (junction 469) -> AAIR.rate_adjust1.decrease2 [order 1] : [copy_Period>rate_period]
      AAIR.rate_adjust1.decrease2 -> (junction 470)
      (junction 469) -> (junction 470) [order 3] : [copy_Period==rate_period]
      (junction 469) -> AAIR.rate_adjust1.increase2 [order 2] : [copy_Period<rate_period]
      AAIR.rate_adjust1.increase2 -> (junction 470)
    AAIR.Pacing1 -> (junction 602) [commented out] : [after(Atr_PW, msec)]
    (junction 603) -> AAIR.Charging_sensing1 [commented out]
    (default) -> AAIR.Rate_adjust.decrease [commented out] : [copy_Period>rate_period]
    (default) -> AAIR.Rate_adjust.increase [commented out] : [copy_Period<rate_period]
    (default) -> AAIR.Rate_adjust [commented out] : [copy_Period==rate_period]
    (default) -> AAIR.INIT1 [commented out]
    AAIR.Pacing -> (junction 455) : [after(Atr_PW, msec)]
    (junction 461) -> AAIR.Charging_sensing
    (junction 470) -> AAIR.ARP_ON
    (junction 539) -> AAIR.ARP_ON
    (junction 590) -> AAIR.ARP_ON1 [commented out]
    (default) -> AAIR.INIT
    AAIR.INIT1 -> AAIR.Charging_sensing1 [commented out]
    (junction 615) -> AAIR.Pacing1 [commented out] : [after(copy_Period-Atr_PW ,msec)]
    AAIR.Charging_sensing1 -> (junction 635) [commented out] : [Set_ARP==1]
    (junction 635) -> (junction 615) [commented out] : [after(ARP,msec)]
    AAIR.ARP_ON1 -> AAIR.Charging_sensing1 [commented out]
    (junction 570) -> AAIR.ARP_ON1 [commented out] : [ATR_CMP_DETECT==1]
    (junction 652) -> (junction 533) [order 1] : [Hys==0]
    AAIR.INIT -> AAIR.Charging_sensing
    (junction 533) -> AAIR.Pacing [order 1] : [after(copy_Period-Atr_PW,msec)]
    (junction 533) -> (junction 538) [order 2] : [ATR_CMP_DETECT==1]
    AAIR.Charging_sensing -> (junction 638) [order 2] : [Set_ARP==1]
    (junction 638) -> (junction 652) : [after(ARP,msec)]
    (junction 652) -> (junction 505) [order 2] : [Hys==1]
    AAIR.Charging_sensing1 -> (junction 570) [commented out] : [Set_ARP==0]
    (junction 570) -> AAIR.Pacing1 [commented out] : [after(copy_Period-Atr_PW, msec)]
    (junction 505) -> (junction 469) [order 1] : [ATR_CMP_DETECT==1]
    (junction 615) -> (junction 589) [commented out] : [ATR_CMP_DETECT==1]
    AAIR.Hys_ON -> AAIR.Charging_sensing
    AAIR.ARP_ON -> AAIR.Hys_ON [order 2] : [Hys_on==1]
    (junction 505) -> AAIR.Pacing [order 2] : [after(copy_Period-Atr_PW+single(Hys_delay) ,msec)]
    AAIR.ARP_ON -> AAIR.Charging_sensing [order 1] : [Hys_on==0]
    (junction 339) -> AAIR.ARP_ON [order 1] : [ATR_CMP_DETECT==1]
    (junction 339) -> AAIR.Pacing [order 2] : [after(copy_Period-Atr_PW, msec)]
    AAIR.Charging_sensing -> (junction 339) [order 1] : [Set_ARP==0]
  state VVIR
    state Charging_sensing [commented out]
      entry:
      %sensing
      FRONTEND_CTRL=1
      VENT_CMP_REF_PWM= VENT_SENSITIVITY
      % Charging C22
      ATR_PACE_CTRL = 0
      VENT_PACE_CTRL = 0
      PACING_REF_PWM = Vent_Amp
      PACE_CHARGE_CTRL = 1
      %Discharging C21
      PACE_GND_CTRL = 1
      VENT_PACE_CTRL = 0
      Z_ATR_CTRL = 0
      Z_VENT_CTRL = 0
      ATR_PACE_CTRL = 0
      ATR_GND_CTRL = 0
      VENT_GND_CTRL = 1
    state Pacing [commented out]
      entry:
      % Discharging C22 to C21
      PACE_CHARGE_CTRL = 0
      PACE_GND_CTRL = 1
      ATR_PACE_CTRL = 0
      ATR_GND_CTRL = 0
      Z_VENT_CTRL = 0
      Z_ATR_CTRL = 0
      VENT_GND_CTRL = 0
      VENT_PACE_CTRL = 1
      %Turn on VRP
      Set_VRP=1
    state INIT [commented out]
      entry:
      Set_VRP=0
    state VRP_ON [commented out]
      entry:
      Set_VRP=1
    state rate_adjust
      state decrease2
        entry:
        copy_Period = copy_Period-single(rf_factor)
      state increase2
        entry:
        copy_Period = copy_Period+single(rf_factor)
      (junction 739) -> VVIR.rate_adjust.decrease2 [order 1] : [copy_Period>rate_period]
      VVIR.rate_adjust.decrease2 -> (junction 740)
      (junction 739) -> (junction 740) [order 3] : [copy_Period==rate_period]
      (junction 739) -> VVIR.rate_adjust.increase2 [order 2] : [copy_Period<rate_period]
      VVIR.rate_adjust.increase2 -> (junction 740)
    note: Hys_on is an input data (locally set for testing)
    state hys_check [commented out]
      (junction 753) -> (junction 754) [commented out] : [Hys==1]
      (junction 753) -> ? [commented out] : [Hys==0]
      (junction 754) -> ? [commented out]
    state INIT1
      entry:
      Set_VRP=0
      copy_Period=single(Period)
      Hys=0
      Hys_delay=Hys_Period
      Hys_on=0
    state Pacing1
      entry:
      % Discharging C22 to C21
      PACE_CHARGE_CTRL = 0
      PACE_GND_CTRL = 1
      ATR_PACE_CTRL = 0
      ATR_GND_CTRL = 0
      Z_VENT_CTRL = 0
      Z_ATR_CTRL = 0
      VENT_GND_CTRL = 0
      VENT_PACE_CTRL = 1
      %Turn on VRP
      Set_VRP=1
    state Charging_sensing1
      entry:
      %sensing
      FRONTEND_CTRL=1
      VENT_CMP_REF_PWM= VENT_SENSITIVITY
      % Charging C22
      ATR_PACE_CTRL = 0
      VENT_PACE_CTRL = 0
      PACING_REF_PWM = Vent_Amp
      PACE_CHARGE_CTRL = 1
      %Discharging C21
      PACE_GND_CTRL = 1
      VENT_PACE_CTRL = 0
      Z_ATR_CTRL = 0
      Z_VENT_CTRL = 0
      ATR_PACE_CTRL = 0
      ATR_GND_CTRL = 0
      VENT_GND_CTRL = 1
    state Hys_ON [commented out]
      entry:
      Hys=0
    state rate_adjust2
      state decrease2
        entry:
        copy_Period = copy_Period-single(rf_factor)
      state increase2
        entry:
        copy_Period = copy_Period+single(rf_factor)
      (junction 765) -> VVIR.rate_adjust2.decrease2 [order 1] : [copy_Period>rate_period]
      VVIR.rate_adjust2.decrease2 -> (junction 766)
      (junction 765) -> (junction 766) [order 3] : [copy_Period==rate_period]
      (junction 765) -> VVIR.rate_adjust2.increase2 [order 2] : [copy_Period<rate_period]
      VVIR.rate_adjust2.increase2 -> (junction 766)
    state VRP_ON1
      entry:
      Set_VRP=1
    state rate_adjust1 [commented out]
      state decrease2 [commented out]
        entry:
        copy_Period = copy_Period-rf_factor
      state increase2 [commented out]
        entry:
        copy_Period = copy_Period+rf_factor
      (junction 778) -> VVIR.rate_adjust1.decrease2 [commented out] : [copy_Period>rate_period]
      VVIR.rate_adjust1.decrease2 -> (junction 779) [commented out]
      (junction 778) -> (junction 779) [commented out] : [copy_Period==rate_period]
      (junction 778) -> VVIR.rate_adjust1.increase2 [commented out] : [copy_Period<rate_period]
      VVIR.rate_adjust1.increase2 -> (junction 779) [commented out]
    (default) -> VVIR.INIT [commented out]
    VVIR.Pacing -> VVIR.Charging_sensing [commented out] : after(Vent_PW, msec)
    VVIR.Charging_sensing -> (junction 318) [commented out] : [Set_VRP==1]
    (junction 318) -> (junction 319) [commented out] : after(VRP,msec)
    (junction 319) -> VVIR.Pacing [commented out] : after(Period-Vent_PW-VRP, msec)
    (junction 319) -> VVIR.VRP_ON [commented out] : [VENT_CMP_DETECT==1]
    VVIR.INIT -> VVIR.Charging_sensing [commented out]
    VVIR.VRP_ON -> VVIR.Charging_sensing [commented out]
    (junction 320) -> VVIR.VRP_ON [commented out] : [VENT_CMP_DETECT==1]
    VVIR.Pacing1 -> (junction 739) : [after(Vent_PW, msec)]
    (junction 791) -> (junction 765) [order 2] : [VENT_CMP_DETECT==1]
    (junction 804) -> (junction 778) [commented out] : [VENT_CMP_DETECT==1]
    VVIR.Charging_sensing -> (junction 320) [commented out] : [Set_VRP==0]
    (junction 320) -> VVIR.Pacing [commented out] : after(Period-Vent_PW, msec)
    (junction 740) -> VVIR.Charging_sensing1
    (junction 766) -> VRP_ON1
    (junction 779) -> VRP_ON1 [commented out]
    (default) -> VVIR.INIT1
    VVIR.INIT1 -> VVIR.Charging_sensing1
    (junction 791) -> VVIR.Pacing1 [order 1] : after((single(copy_Period)-Vent_PW-single(VRP)),msec)
    (junction 803) -> (junction 791) : after(VRP,msec)
    VVIR.Charging_sensing1 -> (junction 803) [order 2] : [Set_VRP==1]
    (junction 821) -> (junction 804) [commented out] : [Hys==1]
    VVIR.Hys_ON -> VVIR.Charging_sensing1 [commented out]
    VRP_ON1 -> VVIR.Hys_ON [commented out] : [Hys_on==1]
    (junction 804) -> VVIR.Pacing1 [commented out] : [after(copy_Period-Vent_PW+Hys_delay ,msec)]
    VRP_ON1 -> VVIR.Charging_sensing1 : [Hys_on==0]
    (junction 797) -> VRP_ON1 [order 1] : [VENT_CMP_DETECT==1]
    (junction 797) -> VVIR.Pacing1 [order 2] : [after(single(copy_Period)-Vent_PW, msec)]
    VVIR.Charging_sensing1 -> (junction 797) [order 1] : [Set_VRP==0]
  state VVI
    state Charging_sensing
      entry:
      %sensing
      FRONTEND_CTRL=1
      VENT_CMP_REF_PWM= VENT_SENSITIVITY
      % Charging C22
      ATR_PACE_CTRL = 0
      VENT_PACE_CTRL = 0
      PACING_REF_PWM = Vent_Amp
      PACE_CHARGE_CTRL = 1
      %Discharging C21
      PACE_GND_CTRL = 1
      VENT_PACE_CTRL = 0
      Z_ATR_CTRL = 0
      Z_VENT_CTRL = 0
      ATR_PACE_CTRL = 0
      ATR_GND_CTRL = 0
      VENT_GND_CTRL = 1
    state Pacing
      entry:
      % Discharging C22 to C21
      PACE_CHARGE_CTRL = 0
      PACE_GND_CTRL = 1
      ATR_PACE_CTRL = 0
      ATR_GND_CTRL = 0
      Z_VENT_CTRL = 0
      Z_ATR_CTRL = 0
      VENT_GND_CTRL = 0
      VENT_PACE_CTRL = 1
      %Turn on VRP
      Set_VRP=1
    state INIT
      entry:
      Set_VRP=0
    state VRP_ON
      entry:
      Set_VRP=1
    (default) -> VVI.INIT
    VVI.Pacing -> VVI.Charging_sensing : after(Vent_PW, msec)
    (junction 229) -> VVI.Pacing [order 1] : after(single(Period)-Vent_PW, msec)
    VVI.Charging_sensing -> (junction 227) [order 1] : [Set_VRP==1]
    (junction 227) -> (junction 229) : after(VRP,msec)
    (junction 229) -> VVI.VRP_ON [order 2] : [VENT_CMP_DETECT==1]
    VVI.INIT -> VVI.Charging_sensing
    VVI.VRP_ON -> VVI.Charging_sensing
    (junction 203) -> VVI.VRP_ON [order 1] : [VENT_CMP_DETECT==1]
    (junction 203) -> VVI.Pacing [order 2] : after(single(Period)-Vent_PW, msec)
    VVI.Charging_sensing -> (junction 203) [order 2] : [Set_VRP==0]
  Mode_Start -> AOOR [order 5] : [Mode==5]
  VOO -> Mode_Start : [Mode ~= 1]
  Mode_Start -> VOO [order 1] : [Mode==1]
  AOOR -> Mode_Start : [Mode ~= 5]
  (default) -> Mode_Start
  Mode_Start -> VOOR [order 6] : [Mode==6]
  VOOR -> Mode_Start : [Mode ~=6]
  Mode_Start -> AAI [order 2] : [Mode==2]
  Mode_Start -> AOO [order 3] : [Mode==3]
  Mode_Start -> AAI [order 9] : [Mode ~= 2]
  AOO -> Mode_Start : [Mode ~= 3]
  DDDR -> Mode_Start [commented out] : [Mode ~= 9]
  Mode_Start -> DDDR [commented out] : [Mode == 9]
  AAIR -> Mode_Start : [Mode~=7]
  Mode_Start -> VVIR [order 8] : [Mode==8]
  VVIR -> Mode_Start : [Mode ~=8]
  Mode_Start -> AAIR [order 7] : [Mode==7]
  VVI -> Mode_Start : [Mode ~=4]
  Mode_Start -> VVI [order 4] : [Mode==4]
  data: rate_period input; rf_factor input; Hys_Period input; Atrial_Amp input; Vent_Amp input; Atr_PW input single; Vent_PW input single; Period input; Mode input; ATR_CMP_DETECT input; VENT_CMP_DETECT input; VRP input uint16; ARP input uint16; ATR_SENSITIVITY input; VENT_SENSITIVITY input; PACE_CHARGE_CTRL output; VENT_CMP_REF_PWM output; Z_ATR_CTRL output; PACING_REF_PWM output; ATR_CMP_REF_PWM output; Z_VENT_CTRL output; ATR_PACE_CTRL output; VENT_PACE_CTRL output; PACE_GND_CTRL output; ATR_GND_CTRL output; VENT_GND_CTRL output; FRONTEND_CTRL output; Hys local; ARP_set local; VRP_set local; Set_VRP local; Set_ARP local; copy_Period local single; Hys_on local; Hys_delay local; Button local; A_Amp local; AV_delay local
